simulink model "fir_simulink_test"  (R2020a)
settings: Solver=VariableStepAuto  StartTime=0.0  StopTime=0.05  RelTol=1e-3
libraries: hdlmdlgenlib x102, dspvision x2
settings Model: Creator=Dell  LastModifiedBy=Dell

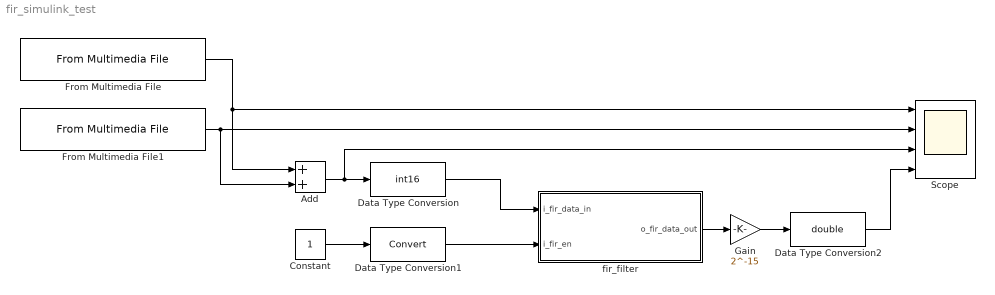
== system fir_simulink_test ==
  Add : Sum
  Constant : Constant  OutDataTypeStr=double  LockScale=on
  Data Type Conversion : DataTypeConversion  OutDataTypeStr=int16  SaturateOnIntegerOverflow=on
  Data Type Conversion1 : DataTypeConversion  SaturateOnIntegerOverflow=on
  Data Type Conversion2 : DataTypeConversion  OutDataTypeStr=double  SaturateOnIntegerOverflow=on
  From Multimedia File : dspvision/From Multimedia File  inputFilename=E:\Designs\Linkedin Projects\resources\project\signal.wav  readRange=[1 inf]  loop=on  numPlays=inf  outputStreams=Audio only  videoDataType=single  audioDataType=double  inheritSampleTime=on  userDefinedSampleTime=1/30  noAudioOutput=off  isIntensityVideo=off  fourcc=RGB  colorVideoFormat=Separate color signals  outputEOF=off  dataOrg=Column-major  audioFrameSize=1  computeAudioFrameSize=off  outSamplingMode=Sample based
  From Multimedia File1 : dspvision/From Multimedia File  inputFilename=E:\Designs\Linkedin Projects\resources\project\noise.wav  readRange=[1 Inf]  loop=on  numPlays=inf  outputStreams=Audio only  videoDataType=single  audioDataType=double  inheritSampleTime=on  userDefinedSampleTime=1/30  noAudioOutput=off  isIntensityVideo=off  fourcc=RGB  colorVideoFormat=Separate color signals  outputEOF=off  dataOrg=Column-major  audioFrameSize=1  computeAudioFrameSize=off  outSamplingMode=Sample based
  Gain : Gain  Gain=2^-15
  Scope : Scope  NumInputPorts=4
  fir_filter : Subsystem
  wires:
  Data Type Conversion/1 -> fir_filter/1(i_fir_data_in)
  Constant/1 -> Data Type Conversion1/1
  Data Type Conversion1/1 -> fir_filter/2(i_fir_en)
  fir_filter/1(o_fir_data_out) -> Gain/1
  Data Type Conversion2/1 -> Scope/4
  From Multimedia File/1 -> Add/1, Scope/1
  From Multimedia File1/1 -> Add/2, Scope/2
  Add/1 -> Data Type Conversion/1, Scope/3
  Gain/1 -> Data Type Conversion2/1

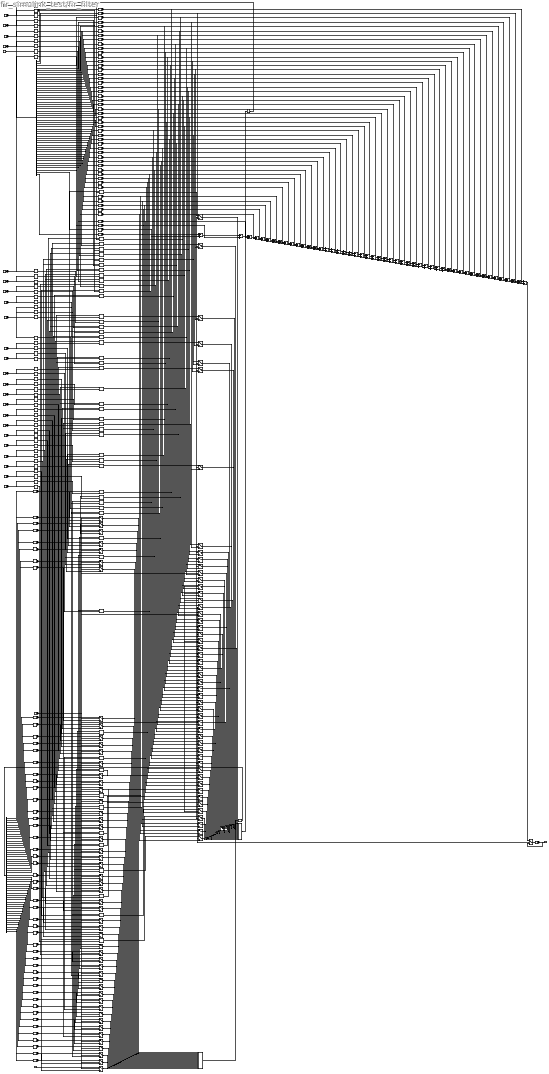
== system fir_simulink_test/fir_filter ==
  i_fir_data_in : Inport  OutDataTypeStr=int16  SampleTime=-1
  i_fir_en : Inport  Port=2  OutDataTypeStr=fixdt(0, 1, 0)  SampleTime=-1
  Add : Sum  AccumDataTypeStr=fixdt(1, 33, 0)  OutDataTypeStr=fixdt(1, 33, 0)  SampleTime=-1
  Add_{1..49} (49 alike) : Sum  AccumDataTypeStr=fixdt(1, 33, 0)  OutDataTypeStr=fixdt(1, 33, 0)  SampleTime=-1
  CONST_u16b_0000000000111110 : Constant  Value=62  OutDataTypeStr=uint16  SampleTime=-1
  CONST_u16b_0000000001010001 : Constant  Value=81  OutDataTypeStr=uint16  SampleTime=-1
  CONST_u16b_0000000010010011 : Constant  Value=147  OutDataTypeStr=uint16  SampleTime=-1
  CONST_u16b_0000000011011010 : Constant  Value=218  OutDataTypeStr=uint16  SampleTime=-1
  CONST_u16b_0000000011011111 : Constant  Value=223  OutDataTypeStr=uint16  SampleTime=-1
  CONST_u16b_0000000011100011 : Constant  Value=227  OutDataTypeStr=uint16  SampleTime=-1
  CONST_u16b_0000000100000010 : Constant  Value=258  OutDataTypeStr=uint16  SampleTime=-1
  CONST_u16b_0000010010000000 : Constant  Value=1152  OutDataTypeStr=uint16  SampleTime=-1
  CONST_u16b_0000100011000111 : Constant  Value=2247  OutDataTypeStr=uint16  SampleTime=-1
  CONST_u16b_0000110100100100 : Constant  Value=3364  OutDataTypeStr=uint16  SampleTime=-1
  CONST_u16b_0001000011101001 : Constant  Value=4329  OutDataTypeStr=uint16  SampleTime=-1
  CONST_u16b_0001001101110111 : Constant  Value=4983  OutDataTypeStr=uint16  SampleTime=-1
  CONST_u16b_0001010001011111 : Constant  Value=5215  OutDataTypeStr=uint16  SampleTime=-1
  CONST_u16b_1111110010111110 : Constant  Value=64702  OutDataTypeStr=uint16  SampleTime=-1
  CONST_u16b_1111110011111101 : Constant  Value=64765  OutDataTypeStr=uint16  SampleTime=-1
  CONST_u16b_1111110101010001 : Constant  Value=64849  OutDataTypeStr=uint16  SampleTime=-1
  CONST_u16b_1111111001010110 : Constant  Value=65110  OutDataTypeStr=uint16  SampleTime=-1
  CONST_u16b_1111111101101110 : Constant  Value=65390  OutDataTypeStr=uint16  SampleTime=-1
  CONST_u16b_1111111111000101 : Constant  Value=65477  OutDataTypeStr=uint16  SampleTime=-1
  CONST_u16b_1111111111001011 : Constant  Value=65483  OutDataTypeStr=uint16  SampleTime=-1
  CONST_u16b_1111111111010010 : Constant  Value=65490  OutDataTypeStr=uint16  SampleTime=-1
  CONST_u16b_1111111111011010 : Constant  Value=65498  OutDataTypeStr=uint16  SampleTime=-1
  CONST_u16b_1111111111101011 : Constant  Value=65515  OutDataTypeStr=uint16  SampleTime=-1
  CONST_u16b_1111111111111010 : Constant  Value=65530  OutDataTypeStr=uint16  SampleTime=-1
  CONST_u16b_1111111111111101 : Constant  Value=65533  OutDataTypeStr=uint16  SampleTime=-1
  Mul : Product  Inputs=**  OutDataTypeStr=fixdt(1, 33, 0)  SampleTime=-1
  Mul_{1..50} (50 alike) : Product  Inputs=**  OutDataTypeStr=fixdt(1, 33, 0)  SampleTime=-1
  Switch : Switch  Criteria=u2 ~= 0  Threshold=double(0)  OutDataTypeStr=int16  SampleTime=-1
  Switch_{1..50} (50 alike) : Switch  Criteria=u2 ~= 0  Threshold=double(0)  OutDataTypeStr=int16  SampleTime=-1
  Switch_{51..102} (52 alike) : Switch  Criteria=u2 ~= 0  Threshold=double(0)  OutDataTypeStr=fixdt(1, 33, 0)  SampleTime=-1
  VectorConcat_1 : Concatenate  NumInputs=51
  VectorConcat_2 : Concatenate  NumInputs=51
  accumulator_FF_0_wire : hdlmdlgenlib/Buffer
      settings: SourceProductBaseCode=SL
  accumulator_FF_10_wire : hdlmdlgenlib/Buffer
      settings: SourceProductBaseCode=SL
  accumulator_FF_11_wire : hdlmdlgenlib/Buffer
      settings: SourceProductBaseCode=SL
  accumulator_FF_12_wire : hdlmdlgenlib/Buffer
      settings: SourceProductBaseCode=SL
  accumulator_FF_13_wire : hdlmdlgenlib/Buffer
      settings: SourceProductBaseCode=SL
  accumulator_FF_14_wire : hdlmdlgenlib/Buffer
      settings: SourceProductBaseCode=SL
  accumulator_FF_15_wire : hdlmdlgenlib/Buffer
      settings: SourceProductBaseCode=SL
  accumulator_FF_16_wire : hdlmdlgenlib/Buffer
      settings: SourceProductBaseCode=SL
  accumulator_FF_17_wire : hdlmdlgenlib/Buffer
      settings: SourceProductBaseCode=SL
  accumulator_FF_18_wire : hdlmdlgenlib/Buffer
      settings: SourceProductBaseCode=SL
  accumulator_FF_19_wire : hdlmdlgenlib/Buffer
      settings: SourceProductBaseCode=SL
  accumulator_FF_1_wire : hdlmdlgenlib/Buffer
      settings: SourceProductBaseCode=SL
  accumulator_FF_20_wire : hdlmdlgenlib/Buffer
      settings: SourceProductBaseCode=SL
  accumulator_FF_21_wire : hdlmdlgenlib/Buffer
      settings: SourceProductBaseCode=SL
  accumulator_FF_22_wire : hdlmdlgenlib/Buffer
      settings: SourceProductBaseCode=SL
  accumulator_FF_23_wire : hdlmdlgenlib/Buffer
      settings: SourceProductBaseCode=SL
  accumulator_FF_24_wire : hdlmdlgenlib/Buffer
      settings: SourceProductBaseCode=SL
  accumulator_FF_25_wire : hdlmdlgenlib/Buffer
      settings: SourceProductBaseCode=SL
  accumulator_FF_26_wire : hdlmdlgenlib/Buffer
      settings: SourceProductBaseCode=SL
  accumulator_FF_27_wire : hdlmdlgenlib/Buffer
      settings: SourceProductBaseCode=SL
  accumulator_FF_28_wire : hdlmdlgenlib/Buffer
      settings: SourceProductBaseCode=SL
  accumulator_FF_29_wire : hdlmdlgenlib/Buffer
      settings: SourceProductBaseCode=SL
  accumulator_FF_2_wire : hdlmdlgenlib/Buffer
      settings: SourceProductBaseCode=SL
  accumulator_FF_30_wire : hdlmdlgenlib/Buffer
      settings: SourceProductBaseCode=SL
  accumulator_FF_31_wire : hdlmdlgenlib/Buffer
      settings: SourceProductBaseCode=SL
  accumulator_FF_32_wire : hdlmdlgenlib/Buffer
      settings: SourceProductBaseCode=SL
  accumulator_FF_33_wire : hdlmdlgenlib/Buffer
      settings: SourceProductBaseCode=SL
  accumulator_FF_34_wire : hdlmdlgenlib/Buffer
      settings: SourceProductBaseCode=SL
  accumulator_FF_35_wire : hdlmdlgenlib/Buffer
      settings: SourceProductBaseCode=SL
  accumulator_FF_36_wire : hdlmdlgenlib/Buffer
      settings: SourceProductBaseCode=SL
  accumulator_FF_37_wire : hdlmdlgenlib/Buffer
      settings: SourceProductBaseCode=SL
  accumulator_FF_38_wire : hdlmdlgenlib/Buffer
      settings: SourceProductBaseCode=SL
  accumulator_FF_39_wire : hdlmdlgenlib/Buffer
      settings: SourceProductBaseCode=SL
  accumulator_FF_3_wire : hdlmdlgenlib/Buffer
      settings: SourceProductBaseCode=SL
  accumulator_FF_40_wire : hdlmdlgenlib/Buffer
      settings: SourceProductBaseCode=SL
  accumulator_FF_41_wire : hdlmdlgenlib/Buffer
      settings: SourceProductBaseCode=SL
  accumulator_FF_42_wire : hdlmdlgenlib/Buffer
      settings: SourceProductBaseCode=SL
  accumulator_FF_43_wire : hdlmdlgenlib/Buffer
      settings: SourceProductBaseCode=SL
  accumulator_FF_44_wire : hdlmdlgenlib/Buffer
      settings: SourceProductBaseCode=SL
  accumulator_FF_45_wire : hdlmdlgenlib/Buffer
      settings: SourceProductBaseCode=SL
  accumulator_FF_46_wire : hdlmdlgenlib/Buffer
      settings: SourceProductBaseCode=SL
  accumulator_FF_47_wire : hdlmdlgenlib/Buffer
      settings: SourceProductBaseCode=SL
  accumulator_FF_48_wire : hdlmdlgenlib/Buffer
      settings: SourceProductBaseCode=SL
  accumulator_FF_49_wire : hdlmdlgenlib/Buffer
      settings: SourceProductBaseCode=SL
  accumulator_FF_4_wire : hdlmdlgenlib/Buffer
      settings: SourceProductBaseCode=SL
  accumulator_FF_50_wire : hdlmdlgenlib/Buffer
      settings: SourceProductBaseCode=SL
  accumulator_FF_5_wire : hdlmdlgenlib/Buffer
      settings: SourceProductBaseCode=SL
  accumulator_FF_6_wire : hdlmdlgenlib/Buffer
      settings: SourceProductBaseCode=SL
  accumulator_FF_7_wire : hdlmdlgenlib/Buffer
      settings: SourceProductBaseCode=SL
  accumulator_FF_8_wire : hdlmdlgenlib/Buffer
      settings: SourceProductBaseCode=SL
  accumulator_FF_9_wire : hdlmdlgenlib/Buffer
      settings: SourceProductBaseCode=SL
  accumulator_reg : Delay  DelayLength=double(1)  InitialCondition=0  SampleTime=-1
  buffer_FF_0_wire : hdlmdlgenlib/Buffer
      settings: SourceProductBaseCode=SL
  buffer_FF_10_wire : hdlmdlgenlib/Buffer
      settings: SourceProductBaseCode=SL
  buffer_FF_11_wire : hdlmdlgenlib/Buffer
      settings: SourceProductBaseCode=SL
  buffer_FF_12_wire : hdlmdlgenlib/Buffer
      settings: SourceProductBaseCode=SL
  buffer_FF_13_wire : hdlmdlgenlib/Buffer
      settings: SourceProductBaseCode=SL
  buffer_FF_14_wire : hdlmdlgenlib/Buffer
      settings: SourceProductBaseCode=SL
  buffer_FF_15_wire : hdlmdlgenlib/Buffer
      settings: SourceProductBaseCode=SL
  buffer_FF_16_wire : hdlmdlgenlib/Buffer
      settings: SourceProductBaseCode=SL
  buffer_FF_17_wire : hdlmdlgenlib/Buffer
      settings: SourceProductBaseCode=SL
  buffer_FF_18_wire : hdlmdlgenlib/Buffer
      settings: SourceProductBaseCode=SL
  buffer_FF_19_wire : hdlmdlgenlib/Buffer
      settings: SourceProductBaseCode=SL
  buffer_FF_1_wire : hdlmdlgenlib/Buffer
      settings: SourceProductBaseCode=SL
  buffer_FF_20_wire : hdlmdlgenlib/Buffer
      settings: SourceProductBaseCode=SL
  buffer_FF_21_wire : hdlmdlgenlib/Buffer
      settings: SourceProductBaseCode=SL
  buffer_FF_22_wire : hdlmdlgenlib/Buffer
      settings: SourceProductBaseCode=SL
  buffer_FF_23_wire : hdlmdlgenlib/Buffer
      settings: SourceProductBaseCode=SL
  buffer_FF_24_wire : hdlmdlgenlib/Buffer
      settings: SourceProductBaseCode=SL
  buffer_FF_25_wire : hdlmdlgenlib/Buffer
      settings: SourceProductBaseCode=SL
  buffer_FF_26_wire : hdlmdlgenlib/Buffer
      settings: SourceProductBaseCode=SL
  buffer_FF_27_wire : hdlmdlgenlib/Buffer
      settings: SourceProductBaseCode=SL
  buffer_FF_28_wire : hdlmdlgenlib/Buffer
      settings: SourceProductBaseCode=SL
  buffer_FF_29_wire : hdlmdlgenlib/Buffer
      settings: SourceProductBaseCode=SL
  buffer_FF_2_wire : hdlmdlgenlib/Buffer
      settings: SourceProductBaseCode=SL
  buffer_FF_30_wire : hdlmdlgenlib/Buffer
      settings: SourceProductBaseCode=SL
  buffer_FF_31_wire : hdlmdlgenlib/Buffer
      settings: SourceProductBaseCode=SL
  buffer_FF_32_wire : hdlmdlgenlib/Buffer
      settings: SourceProductBaseCode=SL
  buffer_FF_33_wire : hdlmdlgenlib/Buffer
      settings: SourceProductBaseCode=SL
  buffer_FF_34_wire : hdlmdlgenlib/Buffer
      settings: SourceProductBaseCode=SL
  buffer_FF_35_wire : hdlmdlgenlib/Buffer
      settings: SourceProductBaseCode=SL
  buffer_FF_36_wire : hdlmdlgenlib/Buffer
      settings: SourceProductBaseCode=SL
  buffer_FF_37_wire : hdlmdlgenlib/Buffer
      settings: SourceProductBaseCode=SL
  buffer_FF_38_wire : hdlmdlgenlib/Buffer
      settings: SourceProductBaseCode=SL
  buffer_FF_39_wire : hdlmdlgenlib/Buffer
      settings: SourceProductBaseCode=SL
  buffer_FF_3_wire : hdlmdlgenlib/Buffer
      settings: SourceProductBaseCode=SL
  buffer_FF_40_wire : hdlmdlgenlib/Buffer
      settings: SourceProductBaseCode=SL
  buffer_FF_41_wire : hdlmdlgenlib/Buffer
      settings: SourceProductBaseCode=SL
  buffer_FF_42_wire : hdlmdlgenlib/Buffer
      settings: SourceProductBaseCode=SL
  buffer_FF_43_wire : hdlmdlgenlib/Buffer
      settings: SourceProductBaseCode=SL
  buffer_FF_44_wire : hdlmdlgenlib/Buffer
      settings: SourceProductBaseCode=SL
  buffer_FF_45_wire : hdlmdlgenlib/Buffer
      settings: SourceProductBaseCode=SL
  buffer_FF_46_wire : hdlmdlgenlib/Buffer
      settings: SourceProductBaseCode=SL
  buffer_FF_47_wire : hdlmdlgenlib/Buffer
      settings: SourceProductBaseCode=SL
  buffer_FF_48_wire : hdlmdlgenlib/Buffer
      settings: SourceProductBaseCode=SL
  buffer_FF_49_wire : hdlmdlgenlib/Buffer
      settings: SourceProductBaseCode=SL
  buffer_FF_4_wire : hdlmdlgenlib/Buffer
      settings: SourceProductBaseCode=SL
  buffer_FF_50_wire : hdlmdlgenlib/Buffer
      settings: SourceProductBaseCode=SL
  buffer_FF_5_wire : hdlmdlgenlib/Buffer
      settings: SourceProductBaseCode=SL
  buffer_FF_6_wire : hdlmdlgenlib/Buffer
      settings: SourceProductBaseCode=SL
  buffer_FF_7_wire : hdlmdlgenlib/Buffer
      settings: SourceProductBaseCode=SL
  buffer_FF_8_wire : hdlmdlgenlib/Buffer
      settings: SourceProductBaseCode=SL
  buffer_FF_9_wire : hdlmdlgenlib/Buffer
      settings: SourceProductBaseCode=SL
  buffer_reg : Delay  DelayLength=double(1)  InitialCondition=0  SampleTime=-1
  dtc{,1..49} (50 alike) : DataTypeConversion  OutDataTypeStr=int16  SampleTime=-1
  o_fir_data_out_1_reg : Delay  DelayLength=double(1)  InitialCondition=0  SampleTime=-1
  t : Demux  Outputs=51
  t1 : Demux  Outputs=51
  o_fir_data_out : Outport  OutDataTypeStr=fixdt(1, 33, 0)
  wires:
  t1/51 -> accumulator_FF_50_wire/1
  CONST_u16b_0000000011011111/1 -> dtc40/1, dtc9/1
  t1/50 -> accumulator_FF_49_wire/1
  t1/49 -> accumulator_FF_48_wire/1
  Switch_41/1 -> VectorConcat_1/42
  t1/48 -> accumulator_FF_47_wire/1
  CONST_u16b_0000000011100011/1 -> dtc30/1, dtc19/1
  t1/47 -> accumulator_FF_46_wire/1
  Add_7/1 -> Add_6/1
  t1/46 -> accumulator_FF_45_wire/1
  t1/45 -> accumulator_FF_44_wire/1
  Switch_40/1 -> VectorConcat_1/41
  t1/44 -> accumulator_FF_43_wire/1
  t1/43 -> accumulator_FF_42_wire/1
  t1/39 -> accumulator_FF_38_wire/1
  Switch_4/1 -> VectorConcat_1/5
  t1/40 -> accumulator_FF_39_wire/1
  t1/41 -> accumulator_FF_40_wire/1
  t1/42 -> accumulator_FF_41_wire/1
  t1/35 -> accumulator_FF_34_wire/1
  Switch_39/1 -> VectorConcat_1/40
  Mul_3/1 -> Switch_54/1
  t1/36 -> accumulator_FF_35_wire/1
  t1/37 -> accumulator_FF_36_wire/1
  t1/38 -> accumulator_FF_37_wire/1
  t1/31 -> accumulator_FF_30_wire/1
  Switch_38/1 -> VectorConcat_1/39
  t1/32 -> accumulator_FF_31_wire/1
  t1/33 -> accumulator_FF_32_wire/1
  t1/34 -> accumulator_FF_33_wire/1
  t1/27 -> accumulator_FF_26_wire/1
  Switch_37/1 -> VectorConcat_1/38
  t1/28 -> accumulator_FF_27_wire/1
  t1/29 -> accumulator_FF_28_wire/1
  t1/30 -> accumulator_FF_29_wire/1
  t1/23 -> accumulator_FF_22_wire/1
  Switch_36/1 -> VectorConcat_1/37
  t1/24 -> accumulator_FF_23_wire/1
  t1/25 -> accumulator_FF_24_wire/1
  Add_8/1 -> Add_7/1
  t1/26 -> accumulator_FF_25_wire/1
  t1/19 -> accumulator_FF_18_wire/1
  Switch_35/1 -> VectorConcat_1/36
  t1/20 -> accumulator_FF_19_wire/1
  t1/21 -> accumulator_FF_20_wire/1
  t1/22 -> accumulator_FF_21_wire/1
  t1/15 -> accumulator_FF_14_wire/1
  Switch_34/1 -> VectorConcat_1/35
  Add_26/1 -> Add_25/1
  t1/16 -> accumulator_FF_15_wire/1
  Mul_50/1 -> Switch_101/1
  t1/17 -> accumulator_FF_16_wire/1
  t1/18 -> accumulator_FF_17_wire/1
  t1/11 -> accumulator_FF_10_wire/1
  Switch_33/1 -> VectorConcat_1/34
  t1/12 -> accumulator_FF_11_wire/1
  CONST_u16b_1111111111111010/1 -> dtc43/1, dtc6/1
  t1/13 -> accumulator_FF_12_wire/1
  t1/14 -> accumulator_FF_13_wire/1
  CONST_u16b_1111110010111110/1 -> dtc33/1, dtc16/1
  t1/7 -> accumulator_FF_6_wire/1
  Switch_32/1 -> VectorConcat_1/33
  t1/8 -> accumulator_FF_7_wire/1
  t1/9 -> accumulator_FF_8_wire/1
  CONST_u16b_0001010001011111/1 -> dtc24/1
  t1/10 -> accumulator_FF_9_wire/1
  t1/3 -> accumulator_FF_2_wire/1
  CONST_u16b_0000000010010011/1 -> dtc41/1, dtc8/1
  Switch_31/1 -> VectorConcat_1/32
  t1/4 -> accumulator_FF_3_wire/1
  Add_9/1 -> Add_8/1
  t1/5 -> accumulator_FF_4_wire/1
  t1/6 -> accumulator_FF_5_wire/1
  t/51 -> buffer_FF_50_wire/1
  Add_11/1 -> Add_10/1
  t1/1 -> accumulator_FF_0_wire/1
  t1/2 -> accumulator_FF_1_wire/1
  t/47 -> buffer_FF_46_wire/1
  Switch_3/1 -> VectorConcat_1/4
  t/48 -> buffer_FF_47_wire/1
  i_fir_data_in/1 -> Switch_50/1
  t/49 -> buffer_FF_48_wire/1
  t/50 -> buffer_FF_49_wire/1
  t/43 -> buffer_FF_42_wire/1
  Switch_29/1 -> VectorConcat_1/30
  t/44 -> buffer_FF_43_wire/1
  t/45 -> buffer_FF_44_wire/1
  t/46 -> buffer_FF_45_wire/1
  t/39 -> buffer_FF_38_wire/1
  Switch_28/1 -> VectorConcat_1/29
  t/40 -> buffer_FF_39_wire/1
  t/41 -> buffer_FF_40_wire/1
  t/42 -> buffer_FF_41_wire/1
  t/38 -> buffer_FF_37_wire/1
  t/37 -> buffer_FF_36_wire/1
  Switch_27/1 -> VectorConcat_1/28
  t/36 -> buffer_FF_35_wire/1
  t/35 -> buffer_FF_34_wire/1
  t/34 -> buffer_FF_33_wire/1
  t/33 -> buffer_FF_32_wire/1
  Switch_26/1 -> VectorConcat_1/27
  t/32 -> buffer_FF_31_wire/1
  t/31 -> buffer_FF_30_wire/1
  t/30 -> buffer_FF_29_wire/1
  t/29 -> buffer_FF_28_wire/1
  Switch_25/1 -> VectorConcat_1/26
  t/28 -> buffer_FF_27_wire/1
  Mul_7/1 -> Switch_58/1
  Add_29/1 -> Add_28/1
  t/27 -> buffer_FF_26_wire/1
  Mul_5/1 -> Switch_56/1
  Add_24/1 -> Add_23/1
  t/26 -> buffer_FF_25_wire/1
  t/25 -> buffer_FF_24_wire/1
  Switch_24/1 -> VectorConcat_1/25
  t/24 -> buffer_FF_23_wire/1
  t/23 -> buffer_FF_22_wire/1
  t/22 -> buffer_FF_21_wire/1
  t/21 -> buffer_FF_20_wire/1
  Switch_23/1 -> VectorConcat_1/24
  t/20 -> buffer_FF_19_wire/1
  Mul_45/1 -> Switch_96/1
  Add_21/1 -> Add_20/1
  t/19 -> buffer_FF_18_wire/1
  t/18 -> buffer_FF_17_wire/1
  CONST_u16b_0000010010000000/1 -> dtc29/1, dtc20/1
  t/17 -> buffer_FF_16_wire/1
  CONST_u16b_0001000011101001/1 -> dtc26/1, dtc22/1
  Switch_22/1 -> VectorConcat_1/23
  t/16 -> buffer_FF_15_wire/1
  t/15 -> buffer_FF_14_wire/1
  t/14 -> buffer_FF_13_wire/1
  t/13 -> buffer_FF_12_wire/1
  Switch_21/1 -> VectorConcat_1/22
  t/12 -> buffer_FF_11_wire/1
  t/11 -> buffer_FF_10_wire/1
  t/10 -> buffer_FF_9_wire/1
  t/9 -> buffer_FF_8_wire/1
  Switch_20/1 -> VectorConcat_1/21
  Mul_34/1 -> Switch_85/1
  Add_10/1 -> Add_9/1
  t/8 -> buffer_FF_7_wire/1
  t/7 -> buffer_FF_6_wire/1
  t/6 -> buffer_FF_5_wire/1
  t/5 -> buffer_FF_4_wire/1
  Switch_2/1 -> VectorConcat_1/3
  t/4 -> buffer_FF_3_wire/1
  t/3 -> buffer_FF_2_wire/1
  t/2 -> buffer_FF_1_wire/1
  t/1 -> buffer_FF_0_wire/1
  Add/1 -> Switch_102/1
  Switch_79/1 -> VectorConcat_2/29
  Mul_35/1 -> Switch_86/1
  Add_1/1 -> Add/1
  dtc44/1 -> Mul_5/2
  Add_2/1 -> Add_1/1
  Add_3/1 -> Add_2/1
  Add_4/1 -> Add_3/1
  Add_5/1 -> Add_4/1
  dtc2/1 -> Mul_48/2
  Add_6/1 -> Add_5/1
  dtc40/1 -> Mul_9/2
  Add_12/1 -> Add_11/1
  dtc30/1 -> Mul_19/2
  Mul_39/1 -> Switch_90/1
  Add_13/1 -> Add_12/1
  accumulator_FF_0_wire/1 -> Add/2, Switch_51/3
  Mul_38/1 -> Switch_89/1
  Add_14/1 -> Add_13/1
  Add_15/1 -> Add_14/1
  Add_16/1 -> Add_15/1
  Switch_51/1 -> VectorConcat_2/1
  Mul_42/1 -> Switch_93/1
  Add_17/1 -> Add_16/1
  Mul_41/1 -> Switch_92/1
  Add_18/1 -> Add_17/1
  dtc24/1 -> Mul_25/2
  Add_19/1 -> Add_18/1
  accumulator_FF_43_wire/1 -> Add_43/2, Switch_94/3
  Mul_46/1 -> Switch_97/1
  Add_20/1 -> Add_19/1
  Add_22/1 -> Add_21/1
  Add_23/1 -> Add_22/1
  Switch_82/1 -> VectorConcat_2/32
  Mul_49/1 -> Switch_100/1
  Add_25/1 -> Add_24/1
  dtc48/1 -> Mul_1/2
  Add_27/1 -> Add_26/1
  accumulator_FF_47_wire/1 -> Add_47/2, Switch_98/3
  Mul_8/1 -> Switch_59/1
  Add_28/1 -> Add_27/1
  Add_30/1 -> Add_29/1
  Switch_55/1 -> VectorConcat_2/5
  Add_31/1 -> Add_30/1
  Add_32/1 -> Add_31/1
  Add_33/1 -> Add_32/1
  buffer_FF_41_wire/1 -> Mul_41/1, Switch_41/3, Switch_40/1
  Add_34/1 -> Add_33/1
  Add_35/1 -> Add_34/1
  dtc12/1 -> Mul_38/2
  Add_36/1 -> Add_35/1
  Switch_95/1 -> VectorConcat_2/45
  Add_37/1 -> Add_36/1
  Add_38/1 -> Add_37/1
  Switch_57/1 -> VectorConcat_2/7
  Add_39/1 -> Add_38/1
  dtc35/1 -> Mul_14/2
  Add_40/1 -> Add_39/1
  buffer_FF_45_wire/1 -> Mul_45/1, Switch_45/3, Switch_44/1
  Add_41/1 -> Add_40/1
  dtc45/1 -> Mul_4/2
  Add_42/1 -> Add_41/1
  accumulator_FF_25_wire/1 -> Add_25/2, Switch_76/3
  Add_43/1 -> Add_42/1
  Add_44/1 -> Add_43/1
  accumulator_FF_35_wire/1 -> Add_35/2, Switch_86/3
  Add_45/1 -> Add_44/1
  Switch_59/1 -> VectorConcat_2/9
  Add_46/1 -> Add_45/1
  Add_47/1 -> Add_46/1
  dtc39/1 -> Mul_10/2
  Add_48/1 -> Add_47/1
  buffer_FF_49_wire/1 -> Mul_49/1, Switch_49/3, Switch_48/1
  Add_49/1 -> Add_48/1
  Switch_101/1 -> VectorConcat_2/51
  Switch_100/1 -> VectorConcat_2/50
  accumulator_FF_7_wire/1 -> Add_7/2, Switch_58/3
  Mul_48/1 -> Switch_99/1
  Switch_99/1 -> VectorConcat_2/49
  Mul_47/1 -> Switch_98/1
  Switch_98/1 -> VectorConcat_2/48
  Switch_97/1 -> VectorConcat_2/47
  Switch_96/1 -> VectorConcat_2/46
  Switch_13/1 -> VectorConcat_1/14
  Mul_44/1 -> Switch_95/1
  Mul_43/1 -> Switch_94/1
  Switch_94/1 -> VectorConcat_2/44
  Switch_93/1 -> VectorConcat_2/43
  Switch_92/1 -> VectorConcat_2/42
  Mul_40/1 -> Switch_91/1
  Switch_91/1 -> VectorConcat_2/41
  Switch_90/1 -> VectorConcat_2/40
  Switch_89/1 -> VectorConcat_2/39
  Switch_11/1 -> VectorConcat_1/12
  Mul_37/1 -> Switch_88/1
  Switch_88/1 -> VectorConcat_2/38
  buffer_FF_10_wire/1 -> Mul_10/1, Switch_10/3, Switch_9/1
  Mul_36/1 -> Switch_87/1
  Switch_87/1 -> VectorConcat_2/37
  Switch_86/1 -> VectorConcat_2/36
  Switch_85/1 -> VectorConcat_2/35
  buffer_FF_28_wire/1 -> Mul_28/1, Switch_28/3, Switch_27/1
  Mul_33/1 -> Switch_84/1
  Switch_84/1 -> VectorConcat_2/34
  Mul_32/1 -> Switch_83/1
  Switch_83/1 -> VectorConcat_2/33
  buffer_FF_47_wire/1 -> Mul_47/1, Switch_47/3, Switch_46/1
  Mul_31/1 -> Switch_82/1
  Mul_30/1 -> Switch_81/1
  Switch_81/1 -> VectorConcat_2/31
  Mul_29/1 -> Switch_80/1
  CONST_u16b_0000110100100100/1 -> dtc27/1, dtc21/1
  Switch_80/1 -> VectorConcat_2/30
  Switch_77/1 -> VectorConcat_2/27
  Mul_28/1 -> Switch_79/1
  Switch_19/1 -> VectorConcat_1/20
  Mul_27/1 -> Switch_78/1
  Switch_78/1 -> VectorConcat_2/28
  buffer_FF_24_wire/1 -> Mul_24/1, Switch_24/3, Switch_23/1
  Mul_26/1 -> Switch_77/1
  Mul_25/1 -> Switch_76/1
  Switch_76/1 -> VectorConcat_2/26
  dtc8/1 -> Mul_42/2
  Mul_24/1 -> Switch_75/1
  Mul_20/1 -> Switch_71/1
  Switch_75/1 -> VectorConcat_2/25
  accumulator_FF_31_wire/1 -> Add_31/2, Switch_82/3
  Mul_23/1 -> Switch_74/1
  Switch_74/1 -> VectorConcat_2/24
  dtc33/1 -> Mul_16/2
  Mul_22/1 -> Switch_73/1
  Switch_73/1 -> VectorConcat_2/23
  accumulator_FF_50_wire/1 -> Add_49/1, Switch_101/3
  Mul_21/1 -> Switch_72/1
  Switch_72/1 -> VectorConcat_2/22
  Switch_71/1 -> VectorConcat_2/21
  Mul_19/1 -> Switch_70/1
  Switch_70/1 -> VectorConcat_2/20
  Mul_18/1 -> Switch_69/1
  Switch_69/1 -> VectorConcat_2/19
  buffer_FF_39_wire/1 -> Mul_39/1, Switch_39/3, Switch_38/1
  Mul_17/1 -> Switch_68/1
  Switch_68/1 -> VectorConcat_2/18
  Mul_16/1 -> Switch_67/1
  Switch_67/1 -> VectorConcat_2/17
  buffer_FF_1_wire/1 -> Mul_1/1, Switch_1/3, Switch/1
  Mul_15/1 -> Switch_66/1
  Switch_66/1 -> VectorConcat_2/16
  dtc1/1 -> Mul_49/2, Mul_29/2
  Mul_14/1 -> Switch_65/1
  Switch_65/1 -> VectorConcat_2/15
  Mul_13/1 -> Switch_64/1
  Switch_64/1 -> VectorConcat_2/14
  Switch_44/1 -> VectorConcat_1/45
  Mul_12/1 -> Switch_63/1
  Switch_63/1 -> VectorConcat_2/13
  Mul_11/1 -> Switch_62/1
  Switch_62/1 -> VectorConcat_2/12
  Mul_10/1 -> Switch_61/1
  Switch_61/1 -> VectorConcat_2/11
  VectorConcat_2/1 -> accumulator_reg/1
  Mul_9/1 -> Switch_60/1
  Switch_60/1 -> VectorConcat_2/10
  Switch_58/1 -> VectorConcat_2/8
  Switch_15/1 -> VectorConcat_1/16
  Mul_6/1 -> Switch_57/1
  Switch_56/1 -> VectorConcat_2/6
  Mul_4/1 -> Switch_55/1
  Switch_54/1 -> VectorConcat_2/4
  Switch_17/1 -> VectorConcat_1/18
  Mul_2/1 -> Switch_53/1
  Switch_53/1 -> VectorConcat_2/3
  Mul_1/1 -> Switch_52/1
  Switch_52/1 -> VectorConcat_2/2
  dtc16/1 -> Mul_34/2
  Mul/1 -> Switch_51/1
  Switch_50/1 -> VectorConcat_1/51
  Switch_49/1 -> VectorConcat_1/50
  Switch_48/1 -> VectorConcat_1/49
  Switch_47/1 -> VectorConcat_1/48
  Switch_46/1 -> VectorConcat_1/47
  Switch_45/1 -> VectorConcat_1/46
  Switch_43/1 -> VectorConcat_1/44
  CONST_u16b_1111110101010001/1 -> dtc34/1, dtc15/1
  Switch_42/1 -> VectorConcat_1/43
  Switch_30/1 -> VectorConcat_1/31
  Switch_18/1 -> VectorConcat_1/19
  Switch_16/1 -> VectorConcat_1/17
  Switch_14/1 -> VectorConcat_1/15
  Switch_12/1 -> VectorConcat_1/13
  Switch_10/1 -> VectorConcat_1/11
  CONST_u16b_0000000001010001/1 -> dtc37/1, dtc12/1
  Switch_9/1 -> VectorConcat_1/10
  Switch_8/1 -> VectorConcat_1/9
  Switch_7/1 -> VectorConcat_1/8
  Switch_6/1 -> VectorConcat_1/7
  Switch_5/1 -> VectorConcat_1/6
  Switch_1/1 -> VectorConcat_1/2
  accumulator_FF_29_wire/1 -> Add_29/2, Switch_80/3
  Switch/1 -> VectorConcat_1/1
  dtc49/1 -> Mul/2
  dtc47/1 -> Mul_2/2
  dtc46/1 -> Mul_3/2
  dtc43/1 -> Mul_6/2
  dtc42/1 -> Mul_7/2
  dtc41/1 -> Mul_8/2
  dtc38/1 -> Mul_11/2
  dtc37/1 -> Mul_12/2
  dtc36/1 -> Mul_13/2
  dtc34/1 -> Mul_15/2
  dtc32/1 -> Mul_17/2
  dtc31/1 -> Mul_18/2
  dtc29/1 -> Mul_20/2
  dtc28/1 -> Mul_21/2
  dtc27/1 -> Mul_22/2
  dtc26/1 -> Mul_23/2
  dtc25/1 -> Mul_24/2
  dtc23/1 -> Mul_26/2
  dtc22/1 -> Mul_27/2
  dtc21/1 -> Mul_28/2
  accumulator_FF_41_wire/1 -> Add_41/2, Switch_92/3
  CONST_u16b_0000100011000111/1 -> dtc28/1
  dtc20/1 -> Mul_30/2
  dtc19/1 -> Mul_31/2
  dtc18/1 -> Mul_32/2
  dtc17/1 -> Mul_33/2
  dtc15/1 -> Mul_35/2
  dtc14/1 -> Mul_36/2
  dtc13/1 -> Mul_37/2
  dtc11/1 -> Mul_39/2
  dtc10/1 -> Mul_40/2
  dtc9/1 -> Mul_41/2
  dtc7/1 -> Mul_43/2
  dtc6/1 -> Mul_44/2
  dtc5/1 -> Mul_45/2
  dtc4/1 -> Mul_46/2
  dtc3/1 -> Mul_47/2
  dtc/1 -> Mul_50/2
  accumulator_reg/1 -> t1/1
  buffer_reg/1 -> t/1
  VectorConcat_1/1 -> buffer_reg/1
  Switch_102/1 -> o_fir_data_out_1_reg/1
  accumulator_FF_49_wire/1 -> Add_49/2, Switch_100/3
  accumulator_FF_48_wire/1 -> Add_48/2, Switch_99/3
  accumulator_FF_46_wire/1 -> Add_46/2, Switch_97/3
  accumulator_FF_45_wire/1 -> Add_45/2, Switch_96/3
  accumulator_FF_44_wire/1 -> Add_44/2, Switch_95/3
  accumulator_FF_42_wire/1 -> Add_42/2, Switch_93/3
  accumulator_FF_40_wire/1 -> Add_40/2, Switch_91/3
  accumulator_FF_39_wire/1 -> Add_39/2, Switch_90/3
  accumulator_FF_38_wire/1 -> Add_38/2, Switch_89/3
  accumulator_FF_37_wire/1 -> Add_37/2, Switch_88/3
  accumulator_FF_36_wire/1 -> Add_36/2, Switch_87/3
  accumulator_FF_34_wire/1 -> Add_34/2, Switch_85/3
  accumulator_FF_33_wire/1 -> Add_33/2, Switch_84/3
  accumulator_FF_32_wire/1 -> Add_32/2, Switch_83/3
  accumulator_FF_30_wire/1 -> Add_30/2, Switch_81/3
  accumulator_FF_28_wire/1 -> Add_28/2, Switch_79/3
  accumulator_FF_27_wire/1 -> Add_27/2, Switch_78/3
  accumulator_FF_26_wire/1 -> Add_26/2, Switch_77/3
  accumulator_FF_24_wire/1 -> Add_24/2, Switch_75/3
  accumulator_FF_23_wire/1 -> Add_23/2, Switch_74/3
  accumulator_FF_22_wire/1 -> Add_22/2, Switch_73/3
  accumulator_FF_21_wire/1 -> Add_21/2, Switch_72/3
  accumulator_FF_20_wire/1 -> Add_20/2, Switch_71/3
  accumulator_FF_19_wire/1 -> Add_19/2, Switch_70/3
  accumulator_FF_18_wire/1 -> Add_18/2, Switch_69/3
  accumulator_FF_17_wire/1 -> Add_17/2, Switch_68/3
  accumulator_FF_16_wire/1 -> Add_16/2, Switch_67/3
  accumulator_FF_15_wire/1 -> Add_15/2, Switch_66/3
  accumulator_FF_14_wire/1 -> Add_14/2, Switch_65/3
  accumulator_FF_13_wire/1 -> Add_13/2, Switch_64/3
  accumulator_FF_12_wire/1 -> Add_12/2, Switch_63/3
  accumulator_FF_11_wire/1 -> Add_11/2, Switch_62/3
  accumulator_FF_10_wire/1 -> Add_10/2, Switch_61/3
  i_fir_en/1 -> Switch_102/2, Switch_101/2, Switch_100/2, Switch_99/2, Switch_98/2, Switch_97/2, Switch_96/2, Switch_95/2, Switch_94/2, Switch_93/2, Switch_92/2, Switch_91/2, Switch_90/2, Switch_89/2, Switch_88/2, Switch_87/2, Switch_86/2, Switch_85/2, Switch_84/2, Switch_83/2, Switch_82/2, Switch_81/2, Switch_80/2, Switch_79/2, Switch_78/2, Switch_77/2, Switch_76/2, Switch_75/2, Switch_74/2, Switch_73/2, Switch_72/2, Switch_71/2, Switch_70/2, Switch_69/2, Switch_68/2, Switch_67/2, Switch_66/2, Switch_65/2, Switch_64/2, Switch_63/2, Switch_62/2, Switch_61/2, Switch_60/2, Switch_59/2, Switch_58/2, Switch_57/2, Switch_56/2, Switch_55/2, Switch_54/2, Switch_53/2, Switch_52/2, Switch_51/2, Switch_50/2, Switch_49/2, Switch_48/2, Switch_47/2, Switch_46/2, Switch_45/2, Switch_44/2, Switch_43/2, Switch_42/2, Switch_41/2, Switch_40/2, Switch_39/2, Switch_38/2, Switch_37/2, Switch_36/2, Switch_35/2, Switch_34/2, Switch_33/2, Switch_32/2, Switch_31/2, Switch_30/2, Switch_29/2, Switch_28/2, Switch_27/2, Switch_26/2, Switch_25/2, Switch_24/2, Switch_23/2, Switch_22/2, Switch_21/2, Switch_20/2, Switch_19/2, Switch_18/2, Switch_17/2, Switch_16/2, Switch_15/2, Switch_14/2, Switch_13/2, Switch_12/2, Switch_11/2, Switch_10/2, Switch_9/2, Switch_8/2, Switch_7/2, Switch_6/2, Switch_5/2, Switch_4/2, Switch_3/2, Switch_2/2, Switch_1/2, Switch/2
  accumulator_FF_9_wire/1 -> Add_9/2, Switch_60/3
  accumulator_FF_8_wire/1 -> Add_8/2, Switch_59/3
  accumulator_FF_6_wire/1 -> Add_6/2, Switch_57/3
  accumulator_FF_5_wire/1 -> Add_5/2, Switch_56/3
  accumulator_FF_4_wire/1 -> Add_4/2, Switch_55/3
  accumulator_FF_3_wire/1 -> Add_3/2, Switch_54/3
  accumulator_FF_2_wire/1 -> Add_2/2, Switch_53/3
  accumulator_FF_1_wire/1 -> Add_1/2, Switch_52/3
  buffer_FF_50_wire/1 -> Mul_50/1, Switch_50/3, Switch_49/1
  buffer_FF_48_wire/1 -> Mul_48/1, Switch_48/3, Switch_47/1
  buffer_FF_46_wire/1 -> Mul_46/1, Switch_46/3, Switch_45/1
  buffer_FF_44_wire/1 -> Mul_44/1, Switch_44/3, Switch_43/1
  buffer_FF_43_wire/1 -> Mul_43/1, Switch_43/3, Switch_42/1
  buffer_FF_42_wire/1 -> Mul_42/1, Switch_42/3, Switch_41/1
  buffer_FF_40_wire/1 -> Mul_40/1, Switch_40/3, Switch_39/1
  buffer_FF_38_wire/1 -> Mul_38/1, Switch_38/3, Switch_37/1
  buffer_FF_37_wire/1 -> Mul_37/1, Switch_37/3, Switch_36/1
  buffer_FF_36_wire/1 -> Mul_36/1, Switch_36/3, Switch_35/1
  buffer_FF_35_wire/1 -> Mul_35/1, Switch_35/3, Switch_34/1
  buffer_FF_34_wire/1 -> Mul_34/1, Switch_34/3, Switch_33/1
  buffer_FF_33_wire/1 -> Mul_33/1, Switch_33/3, Switch_32/1
  buffer_FF_32_wire/1 -> Mul_32/1, Switch_32/3, Switch_31/1
  CONST_u16b_0000000100000010/1 -> dtc39/1, dtc10/1
  buffer_FF_31_wire/1 -> Mul_31/1, Switch_31/3, Switch_30/1
  buffer_FF_30_wire/1 -> Mul_30/1, Switch_30/3, Switch_29/1
  buffer_FF_29_wire/1 -> Mul_29/1, Switch_29/3, Switch_28/1
  buffer_FF_27_wire/1 -> Mul_27/1, Switch_27/3, Switch_26/1
  buffer_FF_26_wire/1 -> Mul_26/1, Switch_26/3, Switch_25/1
  buffer_FF_25_wire/1 -> Mul_25/1, Switch_25/3, Switch_24/1
  buffer_FF_23_wire/1 -> Mul_23/1, Switch_23/3, Switch_22/1
  buffer_FF_22_wire/1 -> Mul_22/1, Switch_22/3, Switch_21/1
  buffer_FF_21_wire/1 -> Mul_21/1, Switch_21/3, Switch_20/1
  buffer_FF_20_wire/1 -> Mul_20/1, Switch_20/3, Switch_19/1
  buffer_FF_19_wire/1 -> Mul_19/1, Switch_19/3, Switch_18/1
  buffer_FF_18_wire/1 -> Mul_18/1, Switch_18/3, Switch_17/1
  buffer_FF_17_wire/1 -> Mul_17/1, Switch_17/3, Switch_16/1
  CONST_u16b_1111111111111101/1 -> dtc49/1, dtc/1
  buffer_FF_16_wire/1 -> Mul_16/1, Switch_16/3, Switch_15/1
  buffer_FF_15_wire/1 -> Mul_15/1, Switch_15/3, Switch_14/1
  buffer_FF_14_wire/1 -> Mul_14/1, Switch_14/3, Switch_13/1
  CONST_u16b_1111110011111101/1 -> dtc32/1, dtc17/1
  buffer_FF_13_wire/1 -> Mul_13/1, Switch_13/3, Switch_12/1
  CONST_u16b_0000000000111110/1 -> dtc42/1, dtc7/1
  buffer_FF_12_wire/1 -> Mul_12/1, Switch_12/3, Switch_11/1
  buffer_FF_11_wire/1 -> Mul_11/1, Switch_11/3, Switch_10/1
  buffer_FF_9_wire/1 -> Mul_9/1, Switch_9/3, Switch_8/1
  CONST_u16b_1111111111011010/1 -> dtc47/1, dtc2/1
  buffer_FF_8_wire/1 -> Mul_8/1, Switch_8/3, Switch_7/1
  CONST_u16b_1111111111001011/1 -> dtc46/1, dtc3/1
  buffer_FF_7_wire/1 -> Mul_7/1, Switch_7/3, Switch_6/1
  buffer_FF_6_wire/1 -> Mul_6/1, Switch_6/3, Switch_5/1
  buffer_FF_5_wire/1 -> Mul_5/1, Switch_5/3, Switch_4/1
  buffer_FF_4_wire/1 -> Mul_4/1, Switch_4/3, Switch_3/1
  buffer_FF_3_wire/1 -> Mul_3/1, Switch_3/3, Switch_2/1
  buffer_FF_2_wire/1 -> Mul_2/1, Switch_2/3, Switch_1/1
  buffer_FF_0_wire/1 -> Mul/1, Switch/3
  CONST_u16b_0001001101110111/1 -> dtc25/1, dtc23/1
  CONST_u16b_1111111001010110/1 -> dtc35/1, dtc31/1, dtc18/1, dtc14/1
  CONST_u16b_1111111101101110/1 -> dtc36/1, dtc13/1
  CONST_u16b_0000000011011010/1 -> dtc38/1, dtc11/1
  CONST_u16b_1111111111010010/1 -> dtc44/1, dtc5/1
  CONST_u16b_1111111111000101/1 -> dtc45/1, dtc4/1
  CONST_u16b_1111111111101011/1 -> dtc48/1, dtc1/1
  o_fir_data_out_1_reg/1 -> Switch_102/3, o_fir_data_out/1
